simulink model "dlo4opt"  (R2025b)
settings: Solver=FixedStepDiscrete  StartTime=0.0  StopTime=1*10^-2  FixedStep=1*10^-9  RelTol=1e-3
libraries: commrandsrc3 x1
settings Model: Creator=Amanullah Bashir  LastModifiedBy=pc

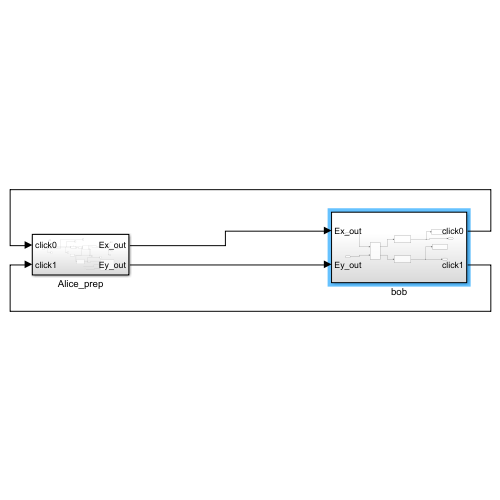
[thumbnail: Simulink's stored preview of the top-level diagram]
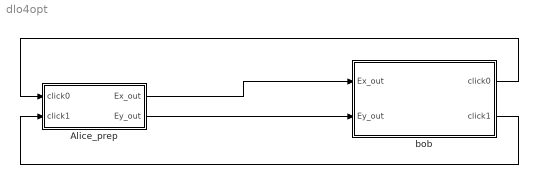
== system dlo4opt ==
  Alice_prep : Subsystem
  bob : Subsystem
  wires:
  Alice_prep/2(Ey_out) -> bob/2(Ey_out)
  Alice_prep/1(Ex_out) -> bob/1(Ex_out)
  bob/1(click0) -> Alice_prep/1(click0)
  bob/2(click1) -> Alice_prep/2(click1)

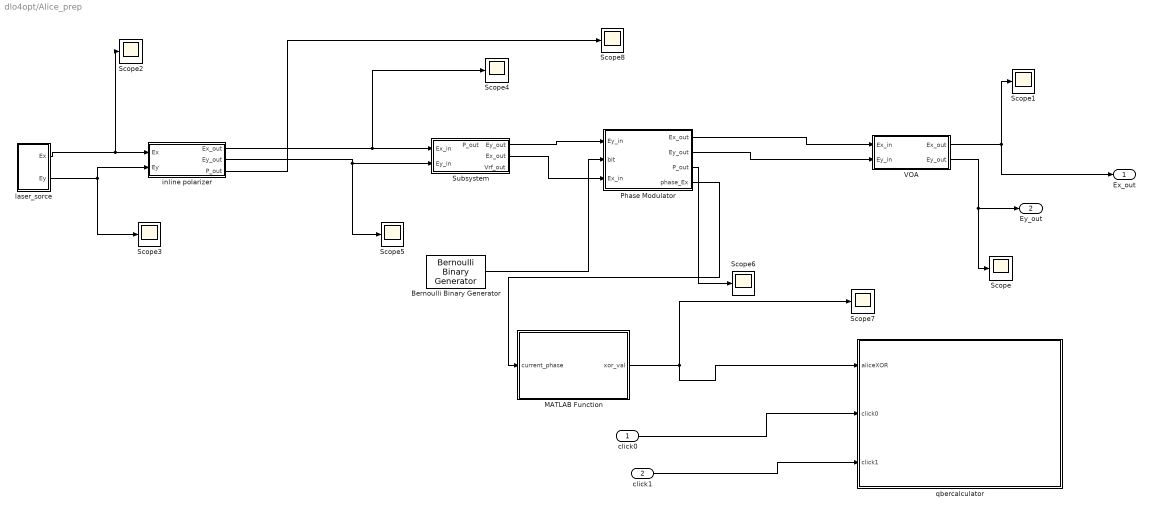
== system dlo4opt/Alice_prep ==
  click0 : Inport
  click1 : Inport  Port=2
  Bernoulli Binary Generator : commrandsrc3/Bernoulli Binary Generator  ProbabilityOfZero=0.5  SeedSource=Auto  Seed=0  SampleTime=1*10^-9  SamplesPerFrame=1  OutputDataType=double  SimulateUsing=Interpreted execution
  MATLAB Function : MATLAB Function  TreatAsAtomicUnit=on
  Phase Modulator : Subsystem
  Scope{,1..8} (9 alike) : Scope
      Scope settings: ActiveDisplayYMinimum=-1  ActiveDisplayYMaximum=1
      Scope1 settings: ActiveDisplayYMinimum=-1  ActiveDisplayYMaximum=1
      Scope2 settings: ActiveDisplayYMinimum=-1E-6  ActiveDisplayYMaximum=7.2E-6
      Scope3 settings: ActiveDisplayYMinimum=-1  ActiveDisplayYMaximum=1  DataLoggingVariableName=ScopeData2
      Scope4 settings: ActiveDisplayYMinimum=-9.2445616507582823E-22  ActiveDisplayYMaximum=3.7067236250439908E-23  DataLoggingVariableName=ScopeData3
      Scope5 settings: ActiveDisplayYMinimum=-1  ActiveDisplayYMaximum=1  DataLoggingVariableName=ScopeData4
      Scope6 settings: ActiveDisplayYMinimum=-6.2764428787815848E-14  ActiveDisplayYMaximum=6.2442909636296011E-14
      Scope7 settings: ActiveDisplayYMinimum=-0.1216403534115208  ActiveDisplayYMaximum=1.1228046362233874  DataLoggingVariableName=ScopeData14
      Scope8 settings: ActiveDisplayYMinimum=-1  ActiveDisplayYMaximum=1  DataLoggingVariableName=ScopeData15
  Subsystem : Subsystem
      settings: PortSchema="{\"entries\":[{\"content\":{\"sides\":[{\"content\":{\"connectorIds\":[\"In1\",\"In2\"]},\"type\":\"ConnectorPlacement.EquallySpacedRectSide\",\"uuid\":\"299cf41b-962f-4f6d-8c66-643055f64068\"},{\"content\":{\"connectorIds\":[\"Out1\",\"Out2\",\"Out3\"],\"side\":\"RIGHT\"},\"type\":\"ConnectorPlacement.EquallySpacedRectSide\",\"uuid\":\"1666e535-aa6a-43b0-baab-95c429bc0632\"},{\"content\":{\"connectorIds\":[\"Out4\"],\"side\":\"TOP\"},\"type\":\"ConnectorPlacement.EquallySpacedRectSide\",\"uuid\":\"42c16f3c-0292-40ec-be3f-efcc357b4ebb\"}]},\"type\":\"ConnectorPlacement.EquallySpacedConnector\",\"uuid\":\"264e6e41-ac9d-4108-acad-5b30193dd194\"}],\"packageUris\":[\"http://schema.mathworks.com/mf0/Connector/R2020b\"],\"version\":\"1.0\"}"
  VOA : Subsystem
  inline polarizer : Subsystem
  laser_sorce : Subsystem
  qbercalculator : Subsystem
  Ex_out : Outport
  Ey_out : Outport  Port=2
  wires:
  laser_sorce/1(Ex) -> Scope2/1, inline polarizer/1(Ex)
  laser_sorce/2(Ey) -> Scope3/1, inline polarizer/2(Ey)
  inline polarizer/1(Ex_out) -> Subsystem/1(Ex_in), Scope4/1
  Phase Modulator/3(P_out) -> Scope6/1
  Phase Modulator/2(Ey_out) -> VOA/2(Ey_in)
  Phase Modulator/1(Ex_out) -> VOA/1(Ex_in)
  VOA/1(Ex_out) -> Ex_out/1, Scope1/1
  VOA/2(Ey_out) -> Scope/1, Ey_out/1
  Bernoulli Binary Generator/1 -> Phase Modulator/2(bit)
  click0/1 -> qbercalculator/2(click0)
  click1/1 -> qbercalculator/3(click1)
  inline polarizer/3(P_out) -> Scope8/1
  Phase Modulator/4(phase_Ex) -> MATLAB Function/1(current_phase)
  inline polarizer/2(Ey_out) -> Scope5/1, Subsystem/2(Ey_in)
  Subsystem/1(Ey_out) -> Phase Modulator/1(Ey_in)
  Subsystem/2(Ex_out) -> Phase Modulator/3(Ex_in)
  MATLAB Function/1(xor_val) -> qbercalculator/1(aliceXOR), Scope7/1

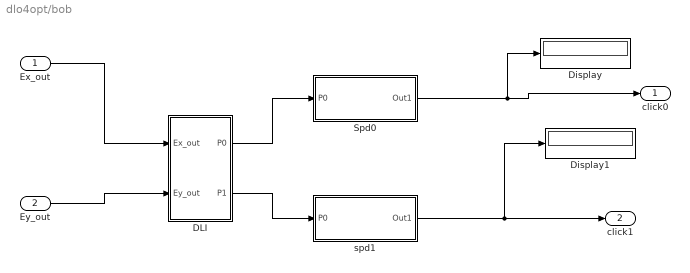
== system dlo4opt/bob ==
  Ex_out : Inport
  Ey_out : Inport  Port=2
  DLI : Subsystem
  Display : Display
  Display1 : Display
  Spd0 : Subsystem
  spd1 : Subsystem
  click0 : Outport
  click1 : Outport  Port=2
  wires:
  Ex_out/1 -> DLI/1(Ex_out)
  Ey_out/1 -> DLI/2(Ey_out)
  DLI/1(P0) -> Spd0/1(P0)
  DLI/2(P1) -> spd1/1(P0)
  spd1/1(Out1) -> Display1/1, click1/1
  Spd0/1(Out1) -> Display/1, click0/1

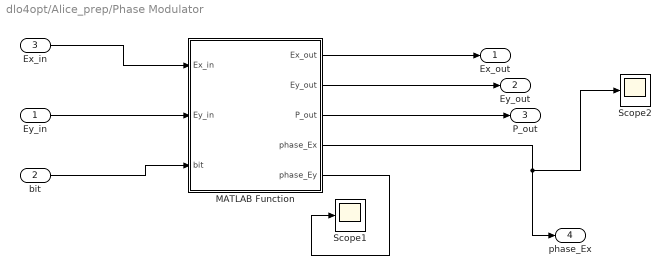
== system dlo4opt/Alice_prep/Phase Modulator ==
  Ey_in : Inport
  bit : Inport  Port=2
  Ex_in : Inport  Port=3
  MATLAB Function : MATLAB Function  TreatAsAtomicUnit=on
  Scope1 : Scope
      settings: ActiveDisplayYMinimum=-3.9269061743732117  ActiveDisplayYMaximum=3.9269424370713337  DataLoggingVariableName=ScopeData5
  Scope2 : Scope
      settings: ActiveDisplayYMinimum=-3.9269061743732117  ActiveDisplayYMaximum=3.9269424370713337  DataLoggingVariableName=ScopeData6
  Ex_out : Outport
  Ey_out : Outport  Port=2
  P_out : Outport  Port=3
  phase_Ex : Outport  Port=4
  wires:
  Ex_in/1 -> MATLAB Function/1(Ex_in)
  Ey_in/1 -> MATLAB Function/2(Ey_in)
  bit/1 -> MATLAB Function/3(bit)
  MATLAB Function/1(Ex_out) -> Ex_out/1
  MATLAB Function/2(Ey_out) -> Ey_out/1
  MATLAB Function/3(P_out) -> P_out/1
  MATLAB Function/4(phase_Ex) -> Scope2/1, phase_Ex/1
  MATLAB Function/5(phase_Ey) -> Scope1/1

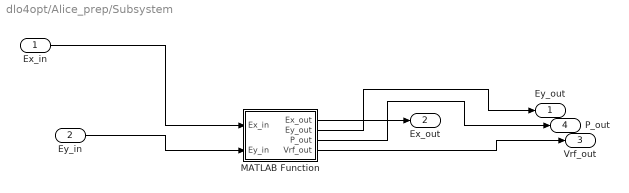
== system dlo4opt/Alice_prep/Subsystem ==
  Ex_in : Inport
  Ey_in : Inport  Port=2
  MATLAB Function : MATLAB Function  TreatAsAtomicUnit=on
  Ey_out : Outport
  Ex_out : Outport  Port=2
  Vrf_out : Outport  Port=3
  P_out : Outport  Port=4
  wires:
  Ey_in/1 -> MATLAB Function/2(Ey_in)
  Ex_in/1 -> MATLAB Function/1(Ex_in)
  MATLAB Function/1(Ex_out) -> Ex_out/1
  MATLAB Function/2(Ey_out) -> Ey_out/1
  MATLAB Function/3(P_out) -> P_out/1
  MATLAB Function/4(Vrf_out) -> Vrf_out/1

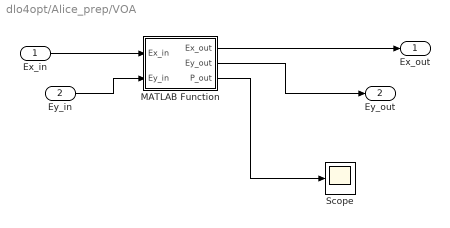
== system dlo4opt/Alice_prep/VOA ==
  Ex_in : Inport
  Ey_in : Inport  Port=2
  MATLAB Function : MATLAB Function  TreatAsAtomicUnit=on
  Scope : Scope
      settings: ActiveDisplayYMinimum=2.824516129032255E-12  ActiveDisplayYMaximum=2.2824516129032267E-11  DataLoggingVariableName=ScopeData7
  Ex_out : Outport
  Ey_out : Outport  Port=2
  wires:
  Ey_in/1 -> MATLAB Function/2(Ey_in)
  MATLAB Function/2(Ey_out) -> Ey_out/1
  Ex_in/1 -> MATLAB Function/1(Ex_in)
  MATLAB Function/1(Ex_out) -> Ex_out/1
  MATLAB Function/3(P_out) -> Scope/1

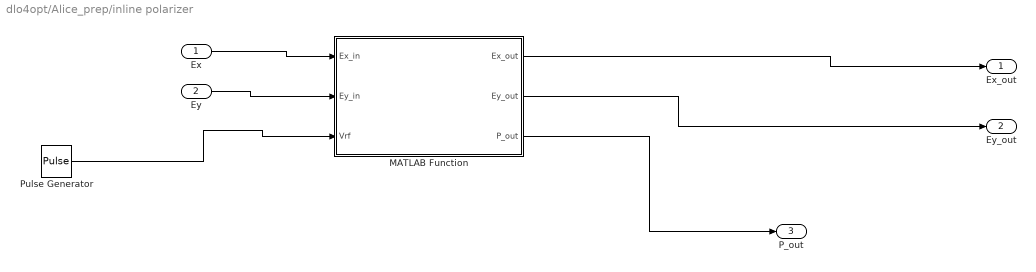
== system dlo4opt/Alice_prep/inline polarizer ==
  Ex : Inport
  Ey : Inport  Port=2
  MATLAB Function : MATLAB Function  TreatAsAtomicUnit=on
  Pulse Generator : DiscretePulseGenerator  Period=10  PulseWidth=3
  Ex_out : Outport
  Ey_out : Outport  Port=2
  P_out : Outport  Port=3
  wires:
  MATLAB Function/1(Ex_out) -> Ex_out/1
  Ex/1 -> MATLAB Function/1(Ex_in)
  Ey/1 -> MATLAB Function/2(Ey_in)
  MATLAB Function/2(Ey_out) -> Ey_out/1
  Pulse Generator/1 -> MATLAB Function/3(Vrf)
  MATLAB Function/3(P_out) -> P_out/1

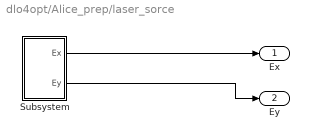
== system dlo4opt/Alice_prep/laser_sorce ==
  Subsystem : Subsystem
  Ex : Outport
  Ey : Outport  Port=2
  wires:
  Subsystem/1(Ex) -> Ex/1
  Subsystem/2(Ey) -> Ey/1

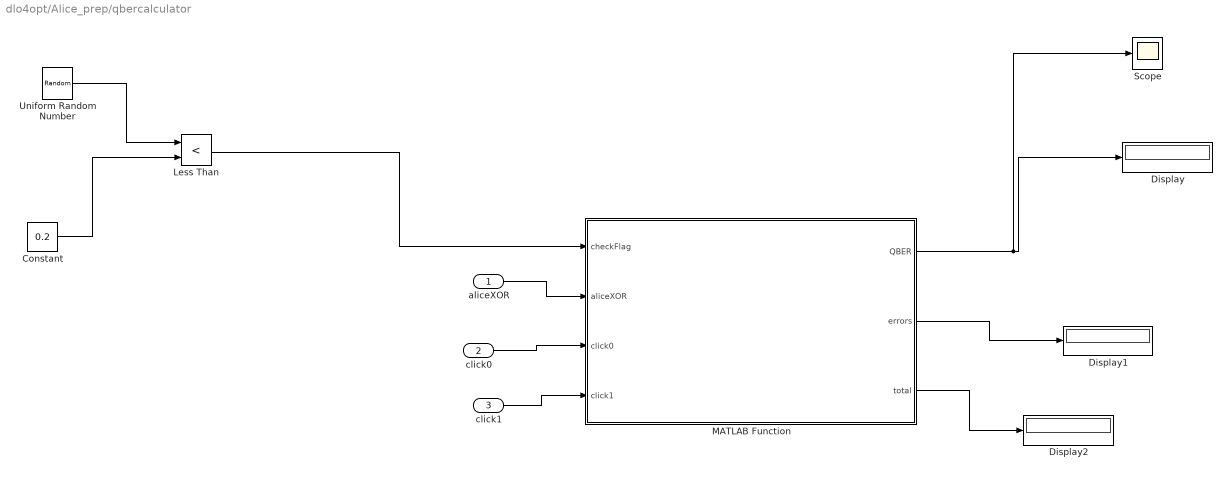
== system dlo4opt/Alice_prep/qbercalculator ==
  aliceXOR : Inport
  click0 : Inport  Port=2
  click1 : Inport  Port=3
  Constant : Constant  Value=0.2
  Display : Display
  Display1 : Display
  Display2 : Display
  Less Than : RelationalOperator  Operator=<  OutDataTypeStr=boolean  RndMeth=Simplest  InputSameDT=off
  MATLAB Function : MATLAB Function  TreatAsAtomicUnit=on
  Scope : Scope
      settings: ActiveDisplayYMinimum=-1  ActiveDisplayYMaximum=1  DataLoggingVariableName=ScopeData17
  Uniform Random Number : UniformRandomNumber  Minimum=0  SampleTime=0.1
  wires:
  aliceXOR/1 -> MATLAB Function/2(aliceXOR)
  click0/1 -> MATLAB Function/3(click0)
  click1/1 -> MATLAB Function/4(click1)
  Uniform Random Number/1 -> Less Than/1
  Constant/1 -> Less Than/2
  Less Than/1 -> MATLAB Function/1(checkFlag)
  MATLAB Function/1(QBER) -> Scope/1, Display/1
  MATLAB Function/2(errors) -> Display1/1
  MATLAB Function/3(total) -> Display2/1

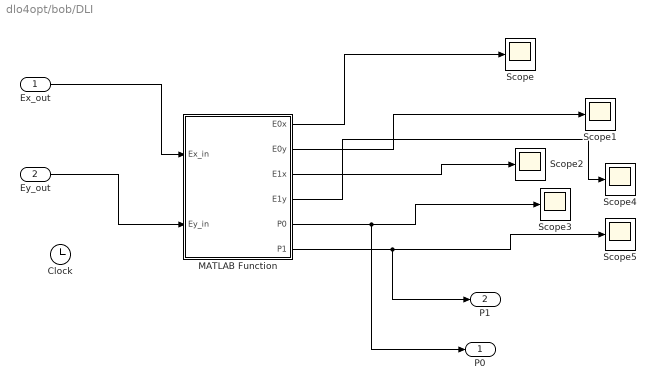
== system dlo4opt/bob/DLI ==
  Ex_out : Inport
  Ey_out : Inport  Port=2
  Clock : Clock
  MATLAB Function : MATLAB Function  TreatAsAtomicUnit=on
  Scope{,1..5} (6 alike) : Scope
      Scope settings: ActiveDisplayYMinimum=-9.5899313805824256E-7  ActiveDisplayYMaximum=1.087693150077201E-6  DataLoggingVariableName=ScopeData8
      Scope1 settings: ActiveDisplayYMinimum=-1  ActiveDisplayYMaximum=1  DataLoggingVariableName=ScopeData9
      Scope2 settings: ActiveDisplayYMinimum=-1.03447430454651E-6  ActiveDisplayYMaximum=1.0286209926541338E-6  DataLoggingVariableName=ScopeData10
      Scope3 settings: ActiveDisplayYMinimum=6.9689844210178346E-13  ActiveDisplayYMaximum=1.8004686454853843E-12  DataLoggingVariableName=ScopeData11
      Scope4 settings: ActiveDisplayYMinimum=-1  ActiveDisplayYMaximum=1  DataLoggingVariableName=ScopeData12
      Scope5 settings: ActiveDisplayYMinimum=6.9689844210178346E-13  ActiveDisplayYMaximum=1.8004686454853843E-12  DataLoggingVariableName=ScopeData13
  P0 : Outport
  P1 : Outport  Port=2
  wires:
  Ex_out/1 -> MATLAB Function/1(Ex_in)
  MATLAB Function/1(E0x) -> Scope/1
  MATLAB Function/2(E0y) -> Scope1/1
  MATLAB Function/3(E1x) -> Scope2/1
  Ey_out/1 -> MATLAB Function/2(Ey_in)
  MATLAB Function/4(E1y) -> Scope4/1
  MATLAB Function/5(P0) -> P0/1, Scope3/1
  MATLAB Function/6(P1) -> P1/1, Scope5/1

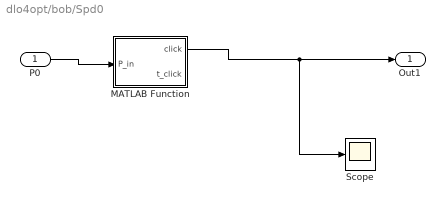
== system dlo4opt/bob/Spd0 ==
  P0 : Inport
  MATLAB Function : MATLAB Function  TreatAsAtomicUnit=on
  Scope : Scope
      settings: ActiveDisplayYMinimum=-0.12499999999999997  ActiveDisplayYMaximum=1.125  DataLoggingVariableName=ScopeData16
  Out1 : Outport
  wires:
  P0/1 -> MATLAB Function/1(P_in)
  MATLAB Function/1(click) -> Scope/1, Out1/1

== system dlo4opt/bob/spd1 ==
  P0 : Inport
  MATLAB Function : MATLAB Function  TreatAsAtomicUnit=on
  Out1 : Outport
  wires:
  P0/1 -> MATLAB Function/1(P_in)
  MATLAB Function/1(click) -> Out1/1

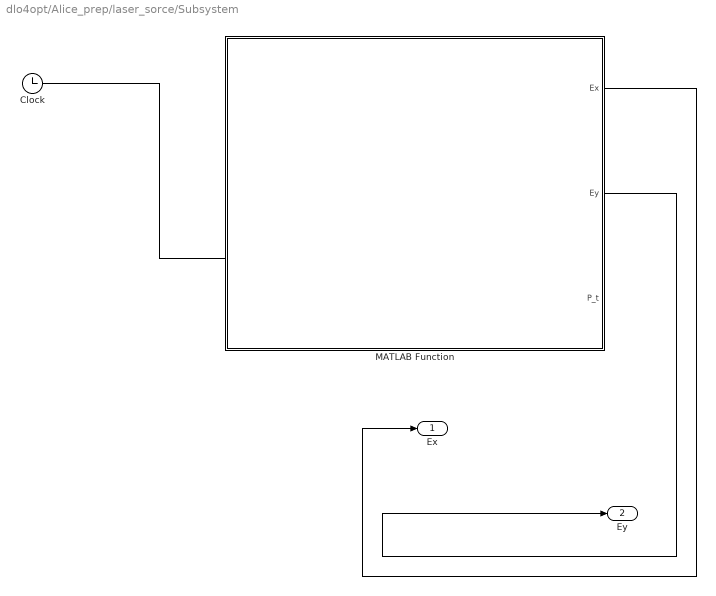
== system dlo4opt/Alice_prep/laser_sorce/Subsystem ==
  Clock : Clock
  MATLAB Function : MATLAB Function  TreatAsAtomicUnit=on
  Ex : Outport
  Ey : Outport  Port=2
  wires:
  MATLAB Function/2(Ey) -> Ey/1
  MATLAB Function/1(Ex) -> Ex/1
  Clock/1 -> ?

== matlab function dlo4opt/Alice_prep/Subsystem/MATLAB Function ==
  data: Ex_in input; Ex_out output; Ey_in input; Ey_out output; P_out output; Vrf_out output

function [Ex_out, Ey_out, P_out, Vrf_out] = im_mzi_auto(Ex_in, Ey_in)
%#codegen
% Self-contained Mach–Zehnder Intensity Modulator for QSDC
% Takes Ex_in, Ey_in from inline polarizer and internally generates RF drive.
% Outputs modulated fields and instantaneous power.

% ---- Device parameters (from paper Table 6) ----
Vpi    = 1.0;      % V (π phase shift voltage)
IL_dB  = 3.0;      % dB insertion loss
Vdc    = 0.5;      % V (quadrature bias = Vpi/2)

% ---- RF generation (Bernoulli random pulses) ----
persistent rngSeeded
if isempty(rngSeeded)
    rng(12345); % deterministic seed for repeatability
    rngSeeded = true;
end

p_on  = 0.5;       % probability of ON
V_on  = 0.5;       % V (ON state)
V_off = 0.0;       % V (OFF state)

if rand < p_on
    Vrf_out = V_on;
else
    Vrf_out = V_off;
end

% ---- Field insertion loss ----
T_field = 10^(-IL_dB/20);

% ---- Transfer function ----
H = T_field * cos(pi * (Vdc + Vrf_out) / Vpi);

% ---- Apply modulation ----
Ex_out = H * Ex_in;
Ey_out = H * Ey_in;

% ---- Compute instantaneous power ----
P_out = abs(Ex_out)^2 + abs(Ey_out)^2;
end

== matlab function dlo4opt/Alice_prep/MATLAB Function ==
  data: current_phase input; xor_val output

function xor_val = xor_phase_from_angle(current_phase)
%#codegen
% Computes XOR of current phase (0 or π) with previous phase using double type.

persistent prev_bit
if isempty(prev_bit)
    prev_bit = 0; % initialize as double
end

% Convert phase to bit: 0 for 0 rad, 1 for π rad
current_bit = double(abs(current_phase - pi) < 1e-6); % 0 or 1 as double

% XOR calculation (result as double)
xor_val = double(xor(logical(current_bit), logical(prev_bit)));

% Update previous bit
prev_bit = current_bit;
end

== matlab function dlo4opt/Alice_prep/inline polarizer/MATLAB Function ==
  data: Ex_in input; Ex_out output; Ey_in input; Ey_out output; Vrf input; P_out output
function [Ex_out, Ey_out, P_out] = im_mzi_stream_hard(Ex_in, Ey_in, Vrf)
%#codegen
% Streaming Mach–Zehnder IM (hard-coded).
% E_out = E_in * cos(pi*(Vdc + Vrf)/Vpi) * T_field

% ---- device parameters (paper Table 6) ----
Vpi    = 1.0;        % V
IL_dB  = 3.0;        % dB (power)
Vdc    = 0.5;        % V (quadrature bias = Vpi/2)

% field insertion loss
T_field = 10^(-IL_dB/20);

% amplitude transfer (real)
H = T_field * cos(pi*(Vdc + Vrf)/Vpi);  % π phase flips when H<0 (physical)

% apply
Ex_out = H .* Ex_in;
Ey_out = H .* Ey_in;

% instantaneous power after IM
P_out  = abs(Ex_out).^2 + abs(Ey_out).^2;
end

== matlab function dlo4opt/Alice_prep/laser_sorce/Subsystem/MATLAB Function ==
  data: Ex output; Ey output; P_t output

function [Ex, Ey, P_t] = laser_pulsed_stream_hard()
%#codegen
% DL04 paper-faithful streaming laser source (baseband).
% One sample per step: Ex (complex), Ey (complex), P_t (double).
%
% Defaults from paper: mu=0.1, lambda0=1547.72 nm, f_clock=1 GHz,
% linewidth=1 MHz, RIN=-160 dB/Hz over B_sys=1 GHz.
% Pulsed envelope: Gaussian FWHM=300 ps (set USE_GAUSS=false for 1 ns rect).

persistent init Ts t Trep sigma P0 U sigmaP sigma_phi USE_GAUSS

if isempty(init)
    % ---- physical constants / paper params ----
    h        = 6.62607015e-34;     % J*s
    c        = 299792458;          % m/s
    lambda0  = 1547.72e-9;         % m
    mu       = 0.1;                % photons/pulse
    f_clock  = 1e9;                % Hz
    Trep     = 1/f_clock;          % s
    linewidth= 1e6;                % Hz
    RIN_dBHz = -160;               % dB/Hz
    B_sys    = 1e9;                % Hz

    % ---- simulation step time ----
    Ts = 10e-12;                   % 10 ps (corrected!)
    
    % ---- envelope choice ----
    USE_GAUSS = true;             % true: Gaussian 300 ps FWHM; false: 1 ns rectangle
    if USE_GAUSS
        FWHM = 300e-12;                           % 300 ps
        sigma = FWHM/(2*sqrt(2*log(2)));          % s
        Eph  = h*c/lambda0;
        U    = mu * Eph;                           % J per pulse
        P0   = U / (sigma*sqrt(2*pi));             % W (peak around center)
    else
        tau_p = 1e-9;                              % 1 ns rectangle
        sigma = 0;                                 % not used
        Eph  = h*c/lambda0;
        U    = mu * Eph;
        P0   = U / tau_p;                          % W (plateau)
    end

    % ---- RIN (absolute power std) using average power over period ----
    P_av    = U / Trep;                                                  % W
    RIN_lin = 10^(RIN_dBHz/10);                                          % 1/Hz
    sigmaP  = RIN_lin * B_sys * P_av;                                    % W

    % ---- phase noise per paper (per-sample Gaussian with τ=1/f_clock) ----
    sigma_phi = 2*pi*linewidth*(Trep);                                   % rad

    % init time
    t    = 0.0;

    init = true;
end

% ---- envelope at current time within the period ----
tau = mod(t + Trep/2, Trep) - Trep/2;   % center each 1 ns period at 0
if USE_GAUSS
    g = exp(-0.5 * (tau/sigma)^2);      % Gaussian pulse
else
    tau_p = 1e-9;
    g = double(abs(tau) <= tau_p/2);
end

% ---- power with RIN (apply where light is present) ----
dP  = sigmaP * randn();
P_t = max(0, P0*g + dP*(g>1e-6));       % keep non-negative; gate RIN by pulse

% ---- phase noise (baseband) ----
phi = sigma_phi * randn();              % per-sample jitter per paper

% ---- Jones field (x-pol only here) ----
Eamp = sqrt(P_t);
Ex   = Eamp .* exp(1j*phi);
Ey   = complex(0.0,0.0);

% advance time
t = t + Ts;
end

== matlab function dlo4opt/Alice_prep/VOA/MATLAB Function ==
  data: Ex_in input; Ex_out output; Ey_in input; Ey_out output; P_out output
function [Ex_out, Ey_out, P_out] = voa_mpn_control(Ex_in, Ey_in)
%#codegen
% Variable Optical Attenuator for QSDC
% Adjusts attenuation to achieve target Mean Photon Number (MPN = 0.1)
% Based on DL04 protocol and paper parameters.

% ---- Fixed parameters from paper ----
lambda = 1550e-9;           % wavelength (meters)
pulse_duration = 1e-9;      % pulse width (seconds)
target_MPN = 0.1;           % desired mean photon number

% ---- Physical constants ----
h = 6.626e-34;              % Planck's constant
c = 3e8;                    % speed of light
E_photon = h*c/lambda;      % energy per photon (J)

% ---- Current power ----
P_in = abs(Ex_in).^2 + abs(Ey_in).^2;

% ---- Required power for target MPN ----
P_required = (target_MPN * E_photon) / pulse_duration;

% ---- Attenuation factor ----
if P_in > 0
    atten_factor = sqrt(P_required / P_in);
else
    atten_factor = 1;
end

% ---- Apply attenuation ----
Ex_out = Ex_in * atten_factor;
Ey_out = Ey_in * atten_factor;

% ---- Output power ----
P_out = abs(Ex_out).^2 + abs(Ey_out).^2;
end

== matlab function dlo4opt/Alice_prep/Phase Modulator/MATLAB Function ==
  data: Ex_in input; Ex_out output; Ey_in input; bit input; Ey_out output; P_out output; phase_Ex output; phase_Ey output

function [Ex_out, Ey_out, P_out, phase_Ex, phase_Ey] = phase_modulator(Ex_in, Ey_in, bit)
%#codegen
% Phase Modulator for QSDC (DL04 protocol)
% Applies 0 or π phase shift and insertion loss (2 dB as per paper).

% ---- Device parameter from paper ----
PM_IL_dB = 2.0;                 % insertion loss in dB
T_field = 10^(-PM_IL_dB/20);    % field transmission factor

% ---- Ensure bit is logical 0 or 1 ----
b = logical(round(bit));        % Convert to 0 or 1 robustly

% ---- Phase modulation ----
phi = pi * double(b);           % phase = 0 or π
ejphi = exp(1j * phi);

% ---- Apply phase and insertion loss ----
Ex_out = T_field .* Ex_in .* ejphi;
Ey_out = T_field .* Ey_in .* ejphi;

% ---- Compute power and phases ----
P_out = abs(Ex_out).^2 + abs(Ey_out).^2;
phase_Ex = angle(Ex_out);
phase_Ey = angle(Ey_out);

== matlab function dlo4opt/bob/DLI/MATLAB Function ==
  data: E0x output; E0y output; E1x output; Ex_in input; Ey_in input; E1y output; P0 output; P1 output


function [E0x, E0y, E1x, E1y, P0, P1] = dli_stream_hard(Ex_in, Ey_in)
% Delay Line Interferometer for DL04 QSDC
% Built-in Ts = 10 ps, delay = 1 ns (adjacent pulse)

persistent init tBS rBS T_field Ns buf_x buf_y idx

if isempty(init)
    % ---- constants ----
    Ts = 10e-12;                   % built-in sample time
    T_dli = 1e-9;                  % 1 ns delay
    Ns = max(1, round(T_dli / Ts));% samples for delay

    tBS = 1/sqrt(2);
    rBS = 1/sqrt(2);
    IL_dB = 9.0;                   % insertion loss
    T_field = 10^(-IL_dB/20);

    buf_x = complex(zeros(Ns,1));
    buf_y = complex(zeros(Ns,1));
    idx   = 1;
    init = true;
end

% read delayed sample
Ex_del = buf_x(idx);
Ey_del = buf_y(idx);

% store current input
buf_x(idx) = Ex_in;
buf_y(idx) = Ey_in;

idx = idx + 1;
if idx > Ns, idx = 1; end

% recombine
E0x = T_field * (tBS*Ex_del + 1i*rBS*Ex_in);
E0y = T_field * (tBS*Ey_del + 1i*rBS*Ey_in);
E1x = T_field * (tBS*Ex_in  + 1i*rBS*Ex_del);
E1y = T_field * (tBS*Ey_in  + 1i*rBS*Ey_del);

P0 = abs(E0x).^2 + abs(E0y).^2;
P1 = abs(E1x).^2 + abs(E1y).^2;
end

== matlab function dlo4opt/bob/Spd0/MATLAB Function ==
  data: P_in input; click output; t_click output


function [click, t_click] = SPD_Block(P_in)
%#codegen
% Single-Photon Detector for QSDC optimized for Simulink MATLAB Function block
% Ts is hardwired to 10^-12 s
% Inputs:
%   P_in : instantaneous power (W)
% Outputs:
%   click   : boolean detection event
%   t_click : timestamp (NaN if no click)

persistent init Ts gate_T Eph eta Pd Nb p0 a deadT jitter E_acc t_now n_since dead_until Ns cnt

if isempty(init)
    % ---- Constants ----
    Ts      = 10e-12;          % Hardwired sample time (10^-12 s)
    gate_T  = 1e-9;            % 1 ns gate
    Ns      = round(gate_T / Ts); % samples per gate

    % SPD parameters
    lambda  = 1547.72e-9;      % wavelength (m)
    eta     = 0.10;            % detection efficiency
    Pd      = 1e-5;            % dark count probability per gate
    Nb      = 1e-5;            % background photons per gate
    p0      = 0.0317;          % afterpulse prefactor
    a       = 0.00115;         % afterpulse decay factor
    deadT   = 10e-6;           % 10 µs dead time
    jitter  = 1e-12;           % 1 ps jitter

    % Photon energy
    h       = 6.62607015e-34;
    c       = 299792458;
    Eph     = h*c/lambda;

    % State variables
    E_acc      = 0.0;
    t_now      = 0.0;
    n_since    = inf;
    dead_until = -inf;
    cnt        = 0;

    init = true;
end

% Accumulate energy
E_acc = E_acc + P_in*Ts;
t_now = t_now + Ts;

click   = false;
t_click = NaN;

% Check gate boundary
cnt = cnt + 1;
if cnt >= Ns
    % Photons in gate
    mu_gate = E_acc / Eph;
    mu_eff  = eta * mu_gate;

    % Signal click probability
    Pp = 1 - exp(-mu_eff);

    % Background photons
    Pb = 1 - exp(-eta * Nb);

    % Afterpulsing
    Pap = p0 * exp(-a * max(0,n_since));

    % Union of independent events
    Pclick = Pp + Pap + Pd + Pb ...
           - (Pp*Pap) - (Pap*Pd) - (Pd*Pp) - (Pb*(Pp+Pap+Pd)) ...
           + (Pp*Pap*Pd);

    % Apply dead time
    if t_now < dead_until
        Pclick = 0.0;
    end

    % Draw event
    if rand() < Pclick
        click = true;
        t_click = t_now + jitter*randn();
        dead_until = t_now + deadT;
        n_since    = 0;
    else
        n_since = n_since + 1;
    end

    % Reset gate accumulator
    E_acc = 0.0;
    cnt   = 0;
end
end

== matlab function dlo4opt/bob/spd1/MATLAB Function ==
  data: P_in input; click output; t_click output


function [click, t_click] = SPD_Block(P_in)
%#codegen
% Single-Photon Detector for QSDC optimized for Simulink MATLAB Function block
% Ts is hardwired to 10^-12 s
% Inputs:
%   P_in : instantaneous power (W)
% Outputs:
%   click   : boolean detection event
%   t_click : timestamp (NaN if no click)

persistent init Ts gate_T Eph eta Pd Nb p0 a deadT jitter E_acc t_now n_since dead_until Ns cnt

if isempty(init)
    % ---- Constants ----
    Ts      = 10e-12;          % Hardwired sample time (10^-12 s)
    gate_T  = 1e-9;            % 1 ns gate
    Ns      = round(gate_T / Ts); % samples per gate

    % SPD parameters
    lambda  = 1547.72e-9;      % wavelength (m)
    eta     = 0.10;            % detection efficiency
    Pd      = 1e-5;            % dark count probability per gate
    Nb      = 1e-5;            % background photons per gate
    p0      = 0.0317;          % afterpulse prefactor
    a       = 0.00115;         % afterpulse decay factor
    deadT   = 10e-6;           % 10 µs dead time
    jitter  = 1e-12;           % 1 ps jitter

    % Photon energy
    h       = 6.62607015e-34;
    c       = 299792458;
    Eph     = h*c/lambda;

    % State variables
    E_acc      = 0.0;
    t_now      = 0.0;
    n_since    = inf;
    dead_until = -inf;
    cnt        = 0;

    init = true;
end

% Accumulate energy
E_acc = E_acc + P_in*Ts;
t_now = t_now + Ts;

click   = false;
t_click = NaN;

% Check gate boundary
cnt = cnt + 1;
if cnt >= Ns
    % Photons in gate
    mu_gate = E_acc / Eph;
    mu_eff  = eta * mu_gate;

    % Signal click probability
    Pp = 1 - exp(-mu_eff);

    % Background photons
    Pb = 1 - exp(-eta * Nb);

    % Afterpulsing
    Pap = p0 * exp(-a * max(0,n_since));

    % Union of independent events
    Pclick = Pp + Pap + Pd + Pb ...
           - (Pp*Pap) - (Pap*Pd) - (Pd*Pp) - (Pb*(Pp+Pap+Pd)) ...
           + (Pp*Pap*Pd);

    % Apply dead time
    if t_now < dead_until
        Pclick = 0.0;
    end

    % Draw event
    if rand() < Pclick
        click = true;
        t_click = t_now + jitter*randn();
        dead_until = t_now + deadT;
        n_since    = 0;
    else
        n_since = n_since + 1;
    end

    % Reset gate accumulator
    E_acc = 0.0;
    cnt   = 0;
end
end

== matlab function dlo4opt/Alice_prep/qbercalculator/MATLAB Function ==
  data: checkFlag input; QBER output; aliceXOR input; click0 input; click1 input; errors output; total output

function [QBER, errors, total] = QBER_Block(checkFlag, aliceXOR, click0, click1)
% QBER calculation for DL04 QSDC forward channel

persistent init E T

if isempty(init)
    E = 0; % error count
    T = 0; % total valid checks
    init = true;
end

if checkFlag
    % Initialize variables
    measBit = -1; % default invalid
    valid = false;

    % Determine measured bit
    if click0 && ~click1
        measBit = 0;
        valid = true;
    elseif click1 && ~click0
        measBit = 1;
        valid = true;
    end

    % Update QBER stats
    if valid
        if measBit ~= aliceXOR
            E = E + 1;
        end
        T = T + 1;
    end
end

errors = E;
total  = T;
if T > 0
    QBER = E / T;
else
    QBER = 0;
end
end
